simulink model "controller13_jumping"  (R2023a)
settings: Solver=FixedStepAuto  StartTime=0.0  StopTime=mdl.exe_time  RelTol=1e-3
values from neighbouring files (symbols this model uses):
  ctr2 = ctr    [s1_setup.m]    (also in step1_setup.m; step1_setup_v1.m)
  lut = gen_lut    [s1_setup.m]    (also in thrust2voltage_lut_20230809.mat = ; thrust2voltage_lut_20230829.mat = )
  mdl = make_model(mdl,rsim)    [s1_setup.m]    (also in setup_controller_with_functions.m = make_model(flight_time); step1_setup.m; step1_setup_v1.m = make_model(flight_time,rsim))
undefined symbols (not defined in the file or in its folder): Angle, Axis, DiscIntNeverNeededParam, rjsim, servo_config, Standard_Devices, UDP_Protocol, use_simulation
libraries: simulink x25, sldrtlib x9, robotcorelib x8, dspmathops x3, dspswit3 x2, shared6dofsys x2, dspfdesign x2, sharedtransform x1, sharedutil x1, matrix_library x1, shared6dof x1, simulink_extras x1
(part 3 of 3)

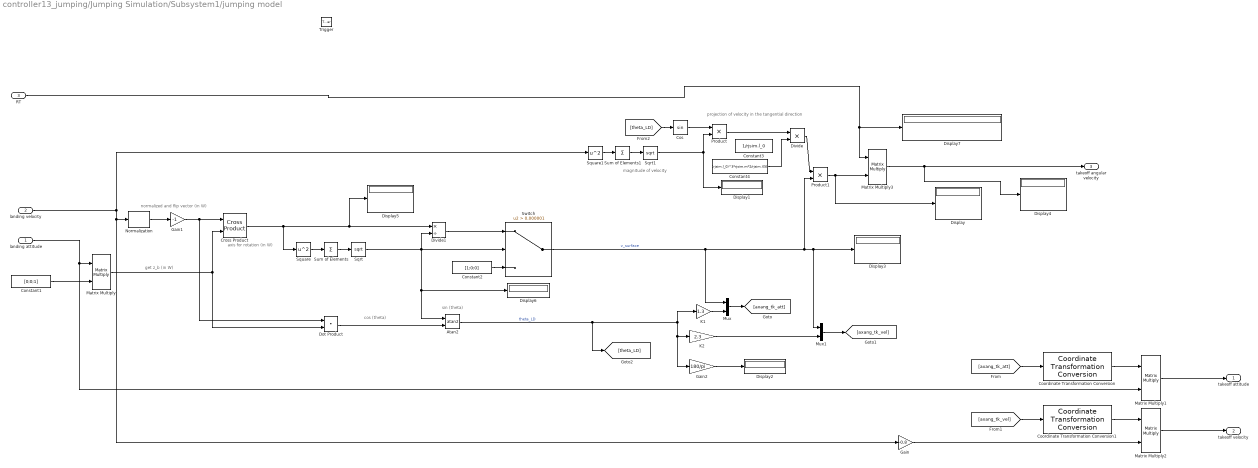
== system controller13_jumping/Jumping Simulation/Subsystem1/jumping model ==
  note: normalized and flip vector (in W)
  note: get z_b (in W)
  note: axis for rotation (in W)
  note: cos (theta)
  note: sin (theta)
  note: magnitude of velocity
  note: projection of velocity in the tangential direction
  landing attitude : Inport
  landing velocity : Inport  Port=2
  RT : Inport  Port=3
  Trigger : TriggerPort  VariantControl=(inherit)
  Atan2 : Trigonometry  Operator=atan2
  Constant1 : Constant  Value=[0;0;1]
  Constant2 : Constant  Value=[1;0;0]
  Constant3 : Constant  Value=1/rjsim.l_0
  Constant4 : Constant  Value=(rjsim.l_0)^3*rjsim.m*2/rjsim.I(5)
  Coordinate Transformation Conversion : robotcorelib/Coordinate Transformation Conversion  InputRepresentation=Axis-Angle  InputEulerSequence=ZYX  ShowTrVecInputPort=on  OutputRepresentation=Rotation Matrix  OutputEulerSequence=ZYX  ShowTrVecOutputPort=on  SimulateUsing=Interpreted execution
      settings: LibrarySourceBlock=navlib/Utilities/Coordinate Transformation Conversion
  Coordinate Transformation Conversion1 : robotcorelib/Coordinate Transformation Conversion  InputRepresentation=Axis-Angle  InputEulerSequence=ZYX  ShowTrVecInputPort=on  OutputRepresentation=Rotation Matrix  OutputEulerSequence=ZYX  ShowTrVecOutputPort=on  SimulateUsing=Interpreted execution
      settings: LibrarySourceBlock=navlib/Utilities/Coordinate Transformation Conversion
  Cos : Trigonometry
  Cross Product : matrix_library/Cross Product
  Display{,1..7} (8 alike) : Display
  Divide : Product  Inputs=**
  Divide1 : Product  Inputs=*/
  Dot Product : DotProduct  OutDataTypeStr=Inherit: Inherit via internal rule
  Gain : Gain  Gain=-0.8
  Gain1 : Gain  Gain=-1
  Gain2 : Gain  Gain=180/pi
  K1 : Gain  Gain=1.3
  K2 : Gain  Gain=2.3
  Matrix Multiply{,1..3} (4 alike) : Product  Multiplication=Matrix(*)
  Mux : Mux  Inputs=2
  Mux1 : Mux  Inputs=2
  Normalization : dspmathops/Normalization  NormType=Squared 2-norm  Bias=1e-10  NormOver=Each column  Dimension=1  roundingMode=Floor  overflowMode=off  accumDataTypeStr=Inherit: Same as product output  accumLastDataTypeStr=Inherit: Same as product output  outputDataTypeStr=Inherit: Same as product output  outputMin=[]  outputMax=[]  outputLastDataTypeStr=Inherit: Same as product output
  Product : Product
  Product1 : Product
  Sqrt : Sqrt
  Sqrt1 : Sqrt
  Square : Math  Operator=square
  Square1 : Math  Operator=square
  Sum of Elements : Sum  Inputs=+
  Sum of Elements1 : Sum  Inputs=+
  Switch : Switch  Criteria=u2 > Threshold  Threshold=0.000001  SaturateOnIntegerOverflow=off  InputSameDT=off
  takeoff attitude : Outport
  takeoff velocity : Outport  Port=2
  takeoff angular velocity : Outport  Port=3
  wires:
  landing velocity/1 -> Gain/1, Normalization/1, Square1/1
  landing attitude/1 -> Matrix Multiply1/2, Matrix Multiply/1
  Constant1/1 -> Matrix Multiply/2
  Normalization/1 -> Gain1/1
  Gain1/1 -> Dot Product/1, Cross Product/1
  Matrix Multiply/1 -> Dot Product/2, Cross Product/2
  Cross Product/1 -> Divide1/1, Display5/1, Square/1
  Square/1 -> Sum of Elements/1
  Sum of Elements/1 -> Sqrt/1
  Sqrt/1 -> Divide1/2, Atan2/1, Display6/1, Switch/2
  Constant2/1 -> Switch/3
  Dot Product/1 -> Atan2/2
  Atan2/1 -> [theta_LD], Gain2/1, K2/1, K1/1  "theta_LD"
  K1/1 -> Mux/2
  Mux/1 -> [axang_tk_att]
  Switch/1 -> Display3/1, Mux1/1, Product1/2, Mux/1  "v_surface"
  Mux1/1 -> [axang_tk_vel]
  K2/1 -> Mux1/2
  Matrix Multiply1/1 -> takeoff attitude/1
  [axang_tk_att] -> Coordinate Transformation Conversion/1
  Coordinate Transformation Conversion/1 -> Matrix Multiply1/1
  [axang_tk_vel] -> Coordinate Transformation Conversion1/1
  Coordinate Transformation Conversion1/1 -> Matrix Multiply2/1
  Gain/1 -> Matrix Multiply2/2
  Matrix Multiply2/1 -> takeoff velocity/1
  Square1/1 -> Sum of Elements1/1
  Sum of Elements1/1 -> Sqrt1/1
  [theta_LD] -> Cos/1
  Cos/1 -> Product/1
  Sqrt1/1 -> Display1/1, Product/2
  Product/1 -> Divide/1
  Divide/1 -> Product1/1
  Product1/1 -> Matrix Multiply3/2, Display/1
  Gain2/1 -> Display2/1
  Divide1/1 -> Switch/1
  RT/1 -> Matrix Multiply3/1, Display7/1
  Matrix Multiply3/1 -> Display4/1, takeoff angular velocity/1
  Constant4/1 -> Divide/2

== system controller13_jumping/Measurement manager 2/safety check system/landing condition ==
  z : Inport
  Add : Sum  Inputs=+--
  SaturatingRamp1 : DiscreteIntegrator  gainval=1  SampleTime=-1  UpperSaturationLimit=1  LowerSaturationLimit=0  ICPrevOutput=DiscIntNeverNeededParam  ICPrevScaledInput=DiscIntNeverNeededParam
  constant : Constant
  constant1 : Constant  Value=2
  constant2 : Constant  Value=mdl.i_delay
  landing_cond : MATLAB Function  TreatAsAtomicUnit=on  SystemSampleTime=mdl.T
  en : Outport
  wires:
  SaturatingRamp1/1 -> Add/1
  constant/1 -> SaturatingRamp1/1
  constant1/1 -> Add/2
  constant2/1 -> Add/3
  Add/1 -> landing_cond/2(time_cond)
  z/1 -> landing_cond/1(alt)
  landing_cond/1(en) -> en/1

== system controller13_jumping/Subsystem6/Subsystem4/If Action Subsystem ==
  In1 : Inport
  In2 : Inport  Port=2
  Action Port : ActionPort  ActionPortLabel=else
  Divide : Product  Inputs=*/
  Out1 : Outport
  wires:
  In1/1 -> Divide/1
  In2/1 -> Divide/2
  Divide/1 -> Out1/1

== system controller13_jumping/Subsystem6/Subsystem4/If Action Subsystem1 ==
  Action Port : ActionPort  ActionPortLabel=if(u1 == 0)
  Constant : Constant  Value=[0;0;0]
  Out1 : Outport
  wires:
  Constant/1 -> Out1/1

== system controller13_jumping/Subsystem6/Subsystem4/Triggered Subsystem ==
  In1 : Inport
  In2 : Inport  Port=2
  Trigger : TriggerPort  VariantControl=(inherit)
  Scope : Scope  NumInputPorts=2
  Timestamp : sldrtlib/Target Profiling/Timestamp
  Unit Delay : UnitDelay  SampleTime=-1  HasFrameUpgradeWarning=on
  Unit Delay1 : UnitDelay  SampleTime=-1  HasFrameUpgradeWarning=on
  Out1 : Outport
  Output : Outport  Port=2
  Output1 : Outport  Port=3
  Output2 : Outport  Port=4
  wires:
  Unit Delay/1 -> Output/1
  Unit Delay1/1 -> Scope/2, Output2/1
  In1/1 -> Unit Delay/1, Out1/1
  In2/1 -> Unit Delay1/1, Scope/1, Output1/1

== system controller13_jumping/Subsystem6/Subsystem5/If Action Subsystem ==
  In1 : Inport
  In2 : Inport  Port=2
  Action Port : ActionPort  ActionPortLabel=else
  Divide : Product  Inputs=*/
  Out1 : Outport
  wires:
  In1/1 -> Divide/1
  In2/1 -> Divide/2
  Divide/1 -> Out1/1

== system controller13_jumping/Subsystem6/Subsystem5/If Action Subsystem1 ==
  Action Port : ActionPort  ActionPortLabel=if(u1 == 0)
  Constant : Constant  Value=zeros(9,1)
  Out1 : Outport
  wires:
  Constant/1 -> Out1/1

== system controller13_jumping/Subsystem6/Subsystem5/Triggered Subsystem ==
  R : Inport
  In2 : Inport  Port=2
  Trigger : TriggerPort  VariantControl=(inherit)
  Scope : Scope  NumInputPorts=2
  Timestamp : sldrtlib/Target Profiling/Timestamp
  Unit Delay : UnitDelay  SampleTime=-1  HasFrameUpgradeWarning=on
  Unit Delay1 : UnitDelay  SampleTime=-1  HasFrameUpgradeWarning=on
  Out1 : Outport
  Output : Outport  Port=2
  Output1 : Outport  Port=3
  Output2 : Outport  Port=4
  wires:
  Unit Delay/1 -> Output/1
  Unit Delay1/1 -> Scope/2, Output2/1
  R/1 -> Unit Delay/1, Out1/1
  In2/1 -> Unit Delay1/1, Scope/1, Output1/1

== system controller13_jumping/signal generator1/Bias_Signal/AveragedBias ==
  note: To avoid having signal "jump",
      | we want SMOOTH transitions
      | in frequency (i.e., a weighted sum
      | of current freq and freq some delta t ago)
  note: time constant = 0.002sec
  In1 : Inport
  Discrete Transfer Fcn : DiscreteTransferFcn  Commented=through  Numerator=[0.05]  Denominator=[1 -.95]
  Out1 : Outport
  wires:
  In1/1 -> Discrete Transfer Fcn/1
  Discrete Transfer Fcn/1 -> Out1/1

== system controller13_jumping/signal generator1/Bias_Signal/SIgnalForRamp_binary ==
  note: Should output 1 or -1,
      | so signal ramps UP to 1
      | or DOWN to 0.
  In1 : Inport
  Add : Sum  Inputs=+-
  Compare To Zero : simulink/Logic and Bit Operations/Compare To Zero  relop=>  OutDataTypeStr=uint8  ZeroCross=off
  Constant : Constant
  Data Type Conversion : DataTypeConversion  OutDataTypeStr=double  SaturateOnIntegerOverflow=off  RndMeth=Floor
  Gain : Gain  Gain=2
  Out1 : Outport
  wires:
  In1/1 -> Compare To Zero/1
  Compare To Zero/1 -> Data Type Conversion/1
  Gain/1 -> Add/1
  Constant/1 -> Add/2
  Add/1 -> Out1/1
  Data Type Conversion/1 -> Gain/1

== system controller13_jumping/signal generator1/Drive_Signal1/AveragedAmp_filtered ==
  note: To avoid having signal "jump",
      | we want SMOOTH transitions
      | in frequency (i.e., a weighted sum
      | of current freq and freq some delta t ago)
  note: time constant 0.002sec
      | for 10kHz samping
  In1 : Inport
  Discrete Transfer Fcn : DiscreteTransferFcn  Commented=through  Numerator=[0.05]  Denominator=[1 -.95]
  Out1 : Outport
  wires:
  In1/1 -> Discrete Transfer Fcn/1
  Discrete Transfer Fcn/1 -> Out1/1

== system controller13_jumping/signal generator1/Drive_Signal1/AveragedOffset_filtered ==
  note: To avoid having signal "jump",
      | we want SMOOTH transitions
      | in frequency (i.e., a weighted sum
      | of current freq and freq some delta t ago)
  note: c
  note: time constant 0.02sec
      | for 10kHz samping
  In1 : Inport
  Discrete Transfer Fcn : DiscreteTransferFcn  Commented=through  Numerator=[0.05]  Denominator=[1 -.95]
  Out1 : Outport
  wires:
  In1/1 -> Discrete Transfer Fcn/1
  Discrete Transfer Fcn/1 -> Out1/1

== system controller13_jumping/signal generator1/Drive_Signal1/AveragedTau_filtered ==
  note: To avoid having signal "jump",
      | we want SMOOTH transitions
      | in frequency (i.e., a weighted sum
      | of current freq and freq some delta t ago)
  note: time constant 0.002sec
      | for 10kHz samping
  In1 : Inport
  Discrete Transfer Fcn : DiscreteTransferFcn  Numerator=[0.05]  Denominator=[1, -0.95]
  Out1 : Outport
  wires:
  In1/1 -> Discrete Transfer Fcn/1
  Discrete Transfer Fcn/1 -> Out1/1

== system controller13_jumping/signal generator1/Drive_Signal1/SignalForRamp_binary ==
  note: Should output 1 or -1,
      | so signal ramps UP to 1
      | or DOWN to 0.
  In1 : Inport
  Add : Sum  Inputs=+-
  Compare To Zero : simulink/Logic and Bit Operations/Compare To Zero  relop=>  OutDataTypeStr=uint8  ZeroCross=off
  Constant : Constant
  Data Type Conversion : DataTypeConversion  OutDataTypeStr=double  SaturateOnIntegerOverflow=off  RndMeth=Floor
  Gain : Gain  Gain=2
  Out1 : Outport
  wires:
  In1/1 -> Compare To Zero/1
  Compare To Zero/1 -> Data Type Conversion/1
  Gain/1 -> Add/1
  Constant/1 -> Add/2
  Add/1 -> Out1/1
  Data Type Conversion/1 -> Gain/1

== system controller13_jumping/signal generator1/Drive_Signal1/SignalForSin_binary ==
  note: We want this to stay "high" for 1
      | second after the actual "enable"
      | is turned off...
  In1 : Inport
  Compare To Zero : simulink/Logic and Bit Operations/Compare To Zero  relop=>  OutDataTypeStr=uint8  ZeroCross=off
  Data Type Conversion : DataTypeConversion  OutDataTypeStr=double  SaturateOnIntegerOverflow=off  RndMeth=Floor
  Out1 : Outport
  wires:
  In1/1 -> Compare To Zero/1
  Compare To Zero/1 -> Data Type Conversion/1
  Data Type Conversion/1 -> Out1/1

== system controller13_jumping/signal generator1/Drive_Signal1/Subsystem ==
  note: positive value pushes the left wing forward
  split cycle mu : Inport
  In2 : Inport  Port=2
  1-mu : Sum  Inputs=+-
  2f : Gain  Gain=2
  2nd harmonic : Trigonometry  OutputSignalType=real
  2pi : Gain  Gain=2*pi
  Abs1 : Abs  SaturateOnIntegerOverflow=off
  Add : Sum
  Constant : Constant
  combined sines : Sum
  deg to rad : Gain  Gain=pi/180
  f : Gain  Gain=-1
  first harmonic : Trigonometry  OutputSignalType=real
  omega*t : DiscreteIntegrator  SampleTime=-1  ICPrevOutput=DiscIntNeverNeededParam  ICPrevScaledInput=DiscIntNeverNeededParam
  phase offset : Constant  Value=0
  signal with gain1 : Product  RndMeth=Zero
  signal with gain2 : Product  RndMeth=Zero
  split cycle signal : Outport
  wires:
  2f/1 -> 2nd harmonic/1
  first harmonic/1 -> signal with gain1/2
  Constant/1 -> 1-mu/1
  split cycle mu/1 -> f/1, Abs1/1
  1-mu/1 -> signal with gain1/1
  2nd harmonic/1 -> signal with gain2/2
  signal with gain1/1 -> combined sines/1
  signal with gain2/1 -> combined sines/2
  combined sines/1 -> split cycle signal/1
  f/1 -> signal with gain2/1
  Abs1/1 -> 1-mu/2
  In2/1 -> 2pi/1
  2pi/1 -> omega*t/1
  omega*t/1 -> Add/2
  Add/1 -> first harmonic/1, 2f/1
  phase offset/1 -> deg to rad/1
  deg to rad/1 -> Add/1

== system controller13_jumping/signal generator1/Drive_Signal2/AveragedAmp_filtered ==
  note: To avoid having signal "jump",
      | we want SMOOTH transitions
      | in frequency (i.e., a weighted sum
      | of current freq and freq some delta t ago)
  note: time constant 0.002sec
      | for 10kHz samping
  In1 : Inport
  Discrete Transfer Fcn : DiscreteTransferFcn  Numerator=[0.05]  Denominator=[1 -.95]
  Out1 : Outport
  wires:
  In1/1 -> Discrete Transfer Fcn/1
  Discrete Transfer Fcn/1 -> Out1/1

== system controller13_jumping/signal generator1/Drive_Signal2/AveragedOffset_filtered ==
  note: To avoid having signal "jump",
      | we want SMOOTH transitions
      | in frequency (i.e., a weighted sum
      | of current freq and freq some delta t ago)
  note: c
  note: time constant 0.02sec
      | for 10kHz samping
  In1 : Inport
  Discrete Transfer Fcn : DiscreteTransferFcn  Numerator=[0.05]  Denominator=[1 -.95]
  Out1 : Outport
  wires:
  In1/1 -> Discrete Transfer Fcn/1
  Discrete Transfer Fcn/1 -> Out1/1

== system controller13_jumping/signal generator1/Drive_Signal2/AveragedTau_filtered ==
  note: To avoid having signal "jump",
      | we want SMOOTH transitions
      | in frequency (i.e., a weighted sum
      | of current freq and freq some delta t ago)
  note: time constant 0.002sec
      | for 10kHz samping
  In1 : Inport
  Discrete Transfer Fcn : DiscreteTransferFcn  Numerator=[0.05]  Denominator=[1, -0.95]
  Out1 : Outport
  wires:
  In1/1 -> Discrete Transfer Fcn/1
  Discrete Transfer Fcn/1 -> Out1/1

== system controller13_jumping/signal generator1/Drive_Signal2/SignalForRamp_binary ==
  note: Should output 1 or -1,
      | so signal ramps UP to 1
      | or DOWN to 0.
  In1 : Inport
  Add : Sum  Inputs=+-
  Compare To Zero : simulink/Logic and Bit Operations/Compare To Zero  relop=>  OutDataTypeStr=uint8  ZeroCross=off
  Constant : Constant
  Data Type Conversion : DataTypeConversion  OutDataTypeStr=double  SaturateOnIntegerOverflow=off  RndMeth=Floor
  Gain : Gain  Gain=2
  Out1 : Outport
  wires:
  In1/1 -> Compare To Zero/1
  Compare To Zero/1 -> Data Type Conversion/1
  Gain/1 -> Add/1
  Constant/1 -> Add/2
  Add/1 -> Out1/1
  Data Type Conversion/1 -> Gain/1

== system controller13_jumping/signal generator1/Drive_Signal2/SignalForSin_binary ==
  note: We want this to stay "high" for 1
      | second after the actual "enable"
      | is turned off...
  In1 : Inport
  Compare To Zero : simulink/Logic and Bit Operations/Compare To Zero  relop=>  OutDataTypeStr=uint8  ZeroCross=off
  Data Type Conversion : DataTypeConversion  OutDataTypeStr=double  SaturateOnIntegerOverflow=off  RndMeth=Floor
  Out1 : Outport
  wires:
  In1/1 -> Compare To Zero/1
  Compare To Zero/1 -> Data Type Conversion/1
  Data Type Conversion/1 -> Out1/1

== system controller13_jumping/signal generator1/Drive_Signal2/Subsystem ==
  note: positive value pushes the left wing forward
  split cycle mu : Inport
  In2 : Inport  Port=2
  1-mu : Sum  Inputs=+-
  2f : Gain  Gain=2
  2nd harmonic : Trigonometry  OutputSignalType=real
  2pi : Gain  Gain=2*pi
  Abs1 : Abs  SaturateOnIntegerOverflow=off
  Add : Sum
  Constant : Constant
  combined sines : Sum
  deg to rad : Gain  Gain=pi/180
  f : Gain  Gain=-1
  first harmonic : Trigonometry  OutputSignalType=real
  omega*t : DiscreteIntegrator  SampleTime=-1  ICPrevOutput=DiscIntNeverNeededParam  ICPrevScaledInput=DiscIntNeverNeededParam
  phase offset : Constant  Value=0
  signal with gain1 : Product  RndMeth=Zero
  signal with gain2 : Product  RndMeth=Zero
  split cycle signal : Outport
  wires:
  2f/1 -> 2nd harmonic/1
  first harmonic/1 -> signal with gain1/2
  Constant/1 -> 1-mu/1
  split cycle mu/1 -> f/1, Abs1/1
  1-mu/1 -> signal with gain1/1
  2nd harmonic/1 -> signal with gain2/2
  signal with gain1/1 -> combined sines/1
  signal with gain2/1 -> combined sines/2
  combined sines/1 -> split cycle signal/1
  f/1 -> signal with gain2/1
  Abs1/1 -> 1-mu/2
  In2/1 -> 2pi/1
  2pi/1 -> omega*t/1
  omega*t/1 -> Add/2
  Add/1 -> first harmonic/1, 2f/1
  phase offset/1 -> deg to rad/1
  deg to rad/1 -> Add/1

== system controller13_jumping/signal generator1/Drive_Signal3/AveragedAmp_filtered ==
  note: To avoid having signal "jump",
      | we want SMOOTH transitions
      | in frequency (i.e., a weighted sum
      | of current freq and freq some delta t ago)
  note: time constant 0.002sec
      | for 10kHz samping
  In1 : Inport
  Discrete Transfer Fcn : DiscreteTransferFcn  Numerator=[0.05]  Denominator=[1 -.95]
  Out1 : Outport
  wires:
  In1/1 -> Discrete Transfer Fcn/1
  Discrete Transfer Fcn/1 -> Out1/1

== system controller13_jumping/signal generator1/Drive_Signal3/AveragedOffset_filtered ==
  note: To avoid having signal "jump",
      | we want SMOOTH transitions
      | in frequency (i.e., a weighted sum
      | of current freq and freq some delta t ago)
  note: c
  note: time constant 0.02sec
      | for 10kHz samping
  In1 : Inport
  Discrete Transfer Fcn : DiscreteTransferFcn  Numerator=[0.05]  Denominator=[1 -.95]
  Out1 : Outport
  wires:
  In1/1 -> Discrete Transfer Fcn/1
  Discrete Transfer Fcn/1 -> Out1/1

== system controller13_jumping/signal generator1/Drive_Signal3/AveragedTau_filtered ==
  note: To avoid having signal "jump",
      | we want SMOOTH transitions
      | in frequency (i.e., a weighted sum
      | of current freq and freq some delta t ago)
  note: time constant 0.002sec
      | for 10kHz samping
  In1 : Inport
  Discrete Transfer Fcn : DiscreteTransferFcn  Numerator=[0.05]  Denominator=[1 -.95]
  Out1 : Outport
  wires:
  In1/1 -> Discrete Transfer Fcn/1
  Discrete Transfer Fcn/1 -> Out1/1

== system controller13_jumping/signal generator1/Drive_Signal3/SignalForRamp_binary ==
  note: Should output 1 or -1,
      | so signal ramps UP to 1
      | or DOWN to 0.
  In1 : Inport
  Add : Sum  Inputs=+-
  Compare To Zero : simulink/Logic and Bit Operations/Compare To Zero  relop=>  OutDataTypeStr=uint8  ZeroCross=off
  Constant : Constant
  Data Type Conversion : DataTypeConversion  OutDataTypeStr=double  SaturateOnIntegerOverflow=off  RndMeth=Floor
  Gain : Gain  Gain=2
  Out1 : Outport
  wires:
  In1/1 -> Compare To Zero/1
  Compare To Zero/1 -> Data Type Conversion/1
  Gain/1 -> Add/1
  Constant/1 -> Add/2
  Add/1 -> Out1/1
  Data Type Conversion/1 -> Gain/1

== system controller13_jumping/signal generator1/Drive_Signal3/SignalForSin_binary ==
  note: We want this to stay "high" for 1
      | second after the actual "enable"
      | is turned off...
  In1 : Inport
  Compare To Zero : simulink/Logic and Bit Operations/Compare To Zero  relop=>  OutDataTypeStr=uint8  ZeroCross=off
  Data Type Conversion : DataTypeConversion  OutDataTypeStr=double  SaturateOnIntegerOverflow=off  RndMeth=Floor
  Out1 : Outport
  wires:
  In1/1 -> Compare To Zero/1
  Compare To Zero/1 -> Data Type Conversion/1
  Data Type Conversion/1 -> Out1/1

== system controller13_jumping/signal generator1/Drive_Signal3/Subsystem ==
  split cycle mu : Inport
  In2 : Inport  Port=2
  1-mu : Sum  Inputs=+-
  2f : Gain  Gain=2
  2nd harmonic : Trigonometry  OutputSignalType=real
  2pi : Gain  Gain=2*pi
  Abs1 : Abs  SaturateOnIntegerOverflow=off
  Constant : Constant
  SmoothClock : DiscreteIntegrator  SampleTime=-1  ICPrevOutput=DiscIntNeverNeededParam  ICPrevScaledInput=DiscIntNeverNeededParam
  combined sines : Sum
  f : Gain
  first harmonic : Trigonometry  OutputSignalType=real
  signal with gain1 : Product  RndMeth=Zero
  signal with gain2 : Product  RndMeth=Zero
  split cycle signal : Outport
  wires:
  SmoothClock/1 -> first harmonic/1, 2f/1
  2f/1 -> 2nd harmonic/1
  2pi/1 -> SmoothClock/1
  first harmonic/1 -> signal with gain1/2
  Constant/1 -> 1-mu/1
  split cycle mu/1 -> f/1, Abs1/1
  1-mu/1 -> signal with gain1/1
  2nd harmonic/1 -> signal with gain2/2
  signal with gain1/1 -> combined sines/1
  signal with gain2/1 -> combined sines/2
  combined sines/1 -> split cycle signal/1
  In2/1 -> 2pi/1
  f/1 -> signal with gain2/1
  Abs1/1 -> 1-mu/2

== system controller13_jumping/signal generator1/Drive_Signal4/AveragedAmp_filtered ==
  note: To avoid having signal "jump",
      | we want SMOOTH transitions
      | in frequency (i.e., a weighted sum
      | of current freq and freq some delta t ago)
  note: time constant 0.002sec
      | for 10kHz samping
  In1 : Inport
  Discrete Transfer Fcn : DiscreteTransferFcn  Commented=through  Numerator=[0.05]  Denominator=[1 -.95]
  Out1 : Outport
  wires:
  In1/1 -> Discrete Transfer Fcn/1
  Discrete Transfer Fcn/1 -> Out1/1

== system controller13_jumping/signal generator1/Drive_Signal4/AveragedOffset_filtered ==
  note: To avoid having signal "jump",
      | we want SMOOTH transitions
      | in frequency (i.e., a weighted sum
      | of current freq and freq some delta t ago)
  note: c
  note: time constant 0.02sec
      | for 10kHz samping
  In1 : Inport
  Discrete Transfer Fcn : DiscreteTransferFcn  Commented=through  Numerator=[0.05]  Denominator=[1 -.95]
  Out1 : Outport
  wires:
  In1/1 -> Discrete Transfer Fcn/1
  Discrete Transfer Fcn/1 -> Out1/1

== system controller13_jumping/signal generator1/Drive_Signal4/AveragedTau_filtered ==
  note: To avoid having signal "jump",
      | we want SMOOTH transitions
      | in frequency (i.e., a weighted sum
      | of current freq and freq some delta t ago)
  note: time constant 0.002sec
      | for 10kHz samping
  In1 : Inport
  Discrete Transfer Fcn : DiscreteTransferFcn  Numerator=[0.05]  Denominator=[1, -0.95]
  Out1 : Outport
  wires:
  In1/1 -> Discrete Transfer Fcn/1
  Discrete Transfer Fcn/1 -> Out1/1

== system controller13_jumping/signal generator1/Drive_Signal4/SignalForRamp_binary ==
  note: Should output 1 or -1,
      | so signal ramps UP to 1
      | or DOWN to 0.
  In1 : Inport
  Add : Sum  Inputs=+-
  Compare To Zero : simulink/Logic and Bit Operations/Compare To Zero  relop=>  OutDataTypeStr=uint8  ZeroCross=off
  Constant : Constant
  Data Type Conversion : DataTypeConversion  OutDataTypeStr=double  SaturateOnIntegerOverflow=off  RndMeth=Floor
  Gain : Gain  Gain=2
  Out1 : Outport
  wires:
  In1/1 -> Compare To Zero/1
  Compare To Zero/1 -> Data Type Conversion/1
  Gain/1 -> Add/1
  Constant/1 -> Add/2
  Add/1 -> Out1/1
  Data Type Conversion/1 -> Gain/1

== system controller13_jumping/signal generator1/Drive_Signal4/SignalForSin_binary ==
  note: We want this to stay "high" for 1
      | second after the actual "enable"
      | is turned off...
  In1 : Inport
  Compare To Zero : simulink/Logic and Bit Operations/Compare To Zero  relop=>  OutDataTypeStr=uint8  ZeroCross=off
  Data Type Conversion : DataTypeConversion  OutDataTypeStr=double  SaturateOnIntegerOverflow=off  RndMeth=Floor
  Out1 : Outport
  wires:
  In1/1 -> Compare To Zero/1
  Compare To Zero/1 -> Data Type Conversion/1
  Data Type Conversion/1 -> Out1/1

== system controller13_jumping/signal generator1/Drive_Signal4/Subsystem ==
  note: positive value pushes the left wing forward
  split cycle mu : Inport
  In2 : Inport  Port=2
  1-mu : Sum  Inputs=+-
  2f : Gain  Gain=2
  2nd harmonic : Trigonometry  OutputSignalType=real
  2pi : Gain  Gain=2*pi
  Abs1 : Abs  SaturateOnIntegerOverflow=off
  Add : Sum
  Constant : Constant
  combined sines : Sum
  deg to rad : Gain  Gain=pi/180
  f : Gain  Gain=-1
  first harmonic : Trigonometry  OutputSignalType=real
  omega*t : DiscreteIntegrator  SampleTime=-1  ICPrevOutput=DiscIntNeverNeededParam  ICPrevScaledInput=DiscIntNeverNeededParam
  phase offset : Constant  Value=0
  signal with gain1 : Product  RndMeth=Zero
  signal with gain2 : Product  RndMeth=Zero
  split cycle signal : Outport
  wires:
  2f/1 -> 2nd harmonic/1
  first harmonic/1 -> signal with gain1/2
  Constant/1 -> 1-mu/1
  split cycle mu/1 -> f/1, Abs1/1
  1-mu/1 -> signal with gain1/1
  2nd harmonic/1 -> signal with gain2/2
  signal with gain1/1 -> combined sines/1
  signal with gain2/1 -> combined sines/2
  combined sines/1 -> split cycle signal/1
  f/1 -> signal with gain2/1
  Abs1/1 -> 1-mu/2
  In2/1 -> 2pi/1
  2pi/1 -> omega*t/1
  omega*t/1 -> Add/2
  Add/1 -> first harmonic/1, 2f/1
  phase offset/1 -> deg to rad/1
  deg to rad/1 -> Add/1

== system controller13_jumping/signal generator1/signal generator 1/SignalForRamp_binary ==
  note: Should output 1 or -1,
      | so signal ramps UP to 1
      | or DOWN to 0.
  EnableSignal : Inport
  Add : Sum  Inputs=+-
  Compare To Zero : simulink/Logic and Bit Operations/Compare To Zero  relop=>  OutDataTypeStr=uint8  ZeroCross=off
  Constant : Constant
  Data Type Conversion : DataTypeConversion  OutDataTypeStr=double  SaturateOnIntegerOverflow=off  RndMeth=Floor
  Gain : Gain  Gain=2
  Out1 : Outport
  wires:
  EnableSignal/1 -> Compare To Zero/1
  Compare To Zero/1 -> Data Type Conversion/1
  Gain/1 -> Add/1
  Constant/1 -> Add/2
  Add/1 -> Out1/1
  Data Type Conversion/1 -> Gain/1

== system controller13_jumping/signal generator1/signal generator 1/SignalSaturationLimit4 ==
  Max : Inport
  SignalRaw : Inport  Port=2
  MaxOf : MinMax  Function=max  Inputs=2
  MinOf : MinMax  Inputs=2
  ground : Constant
  SignalSatd : Outport
  wires:
  SignalRaw/1 -> MinOf/2
  MinOf/1 -> MaxOf/1
  MaxOf/1 -> SignalSatd/1
  Max/1 -> MinOf/1
  ground/1 -> MaxOf/2

== system controller13_jumping/signal generator1/signal generator 1/get max voltage ==
  note: time constant = 0.002sec
  QuasiEnable : Inport
  max voltage : Inport  Port=2
  Product : Product  RndMeth=Zero
  SIgnalForRamp_binary : Subsystem
  SaturatingRamp : DiscreteIntegrator  gainval=100  SampleTime=-1  LimitOutput=on  UpperSaturationLimit=1  LowerSaturationLimit=0  ICPrevOutput=DiscIntNeverNeededParam  ICPrevScaledInput=DiscIntNeverNeededParam
  max signa; : Outport
  wires:
  Product/1 -> max signa;/1
  max voltage/1 -> Product/2
  QuasiEnable/1 -> SIgnalForRamp_binary/1(In1)
  SIgnalForRamp_binary/1(Out1) -> SaturatingRamp/1
  SaturatingRamp/1 -> Product/1

== system controller13_jumping/signal generator1/signal generator 2/SignalForRamp_binary ==
  note: Should output 1 or -1,
      | so signal ramps UP to 1
      | or DOWN to 0.
  EnableSignal : Inport
  Add : Sum  Inputs=+-
  Compare To Zero : simulink/Logic and Bit Operations/Compare To Zero  relop=>  OutDataTypeStr=uint8  ZeroCross=off
  Constant : Constant
  Data Type Conversion : DataTypeConversion  OutDataTypeStr=double  SaturateOnIntegerOverflow=off  RndMeth=Floor
  Gain : Gain  Gain=2
  Out1 : Outport
  wires:
  EnableSignal/1 -> Compare To Zero/1
  Compare To Zero/1 -> Data Type Conversion/1
  Gain/1 -> Add/1
  Constant/1 -> Add/2
  Add/1 -> Out1/1
  Data Type Conversion/1 -> Gain/1

== system controller13_jumping/signal generator1/signal generator 2/SignalSaturationLimit4 ==
  Max : Inport
  SignalRaw : Inport  Port=2
  MaxOf : MinMax  Function=max  Inputs=2
  MinOf : MinMax  Inputs=2
  ground : Constant
  SignalSatd : Outport
  wires:
  SignalRaw/1 -> MinOf/2
  MinOf/1 -> MaxOf/1
  MaxOf/1 -> SignalSatd/1
  Max/1 -> MinOf/1
  ground/1 -> MaxOf/2

== system controller13_jumping/signal generator1/signal generator 2/get max voltage ==
  note: time constant = 0.002sec
  QuasiEnable : Inport
  max voltage : Inport  Port=2
  Product : Product  RndMeth=Zero
  SIgnalForRamp_binary : Subsystem
  SaturatingRamp : DiscreteIntegrator  gainval=100  SampleTime=-1  LimitOutput=on  UpperSaturationLimit=1  LowerSaturationLimit=0  ICPrevOutput=DiscIntNeverNeededParam  ICPrevScaledInput=DiscIntNeverNeededParam
  max signa; : Outport
  wires:
  Product/1 -> max signa;/1
  max voltage/1 -> Product/2
  QuasiEnable/1 -> SIgnalForRamp_binary/1(In1)
  SIgnalForRamp_binary/1(Out1) -> SaturatingRamp/1
  SaturatingRamp/1 -> Product/1

== system controller13_jumping/signal generator1/signal generator 3/SignalForRamp_binary ==
  note: Should output 1 or -1,
      | so signal ramps UP to 1
      | or DOWN to 0.
  EnableSignal : Inport
  Add : Sum  Inputs=+-
  Compare To Zero : simulink/Logic and Bit Operations/Compare To Zero  relop=>  OutDataTypeStr=uint8  ZeroCross=off
  Constant : Constant
  Data Type Conversion : DataTypeConversion  OutDataTypeStr=double  SaturateOnIntegerOverflow=off  RndMeth=Floor
  Gain : Gain  Gain=2
  Out1 : Outport
  wires:
  EnableSignal/1 -> Compare To Zero/1
  Compare To Zero/1 -> Data Type Conversion/1
  Gain/1 -> Add/1
  Constant/1 -> Add/2
  Add/1 -> Out1/1
  Data Type Conversion/1 -> Gain/1

== system controller13_jumping/signal generator1/signal generator 3/SignalSaturationLimit4 ==
  Max : Inport
  SignalRaw : Inport  Port=2
  MaxOf : MinMax  Function=max  Inputs=2
  MinOf : MinMax  Inputs=2
  ground : Constant
  SignalSatd : Outport
  wires:
  SignalRaw/1 -> MinOf/2
  MinOf/1 -> MaxOf/1
  MaxOf/1 -> SignalSatd/1
  Max/1 -> MinOf/1
  ground/1 -> MaxOf/2

== system controller13_jumping/signal generator1/signal generator 3/get max voltage ==
  note: time constant = 0.002sec
  QuasiEnable : Inport
  max voltage : Inport  Port=2
  Product : Product  RndMeth=Zero
  SIgnalForRamp_binary : Subsystem
  SaturatingRamp : DiscreteIntegrator  gainval=100  SampleTime=-1  LimitOutput=on  UpperSaturationLimit=1  LowerSaturationLimit=0  ICPrevOutput=DiscIntNeverNeededParam  ICPrevScaledInput=DiscIntNeverNeededParam
  max signa; : Outport
  wires:
  Product/1 -> max signa;/1
  max voltage/1 -> Product/2
  QuasiEnable/1 -> SIgnalForRamp_binary/1(In1)
  SIgnalForRamp_binary/1(Out1) -> SaturatingRamp/1
  SaturatingRamp/1 -> Product/1

== system controller13_jumping/signal generator1/signal generator 4/SignalForRamp_binary ==
  note: Should output 1 or -1,
      | so signal ramps UP to 1
      | or DOWN to 0.
  EnableSignal : Inport
  Add : Sum  Inputs=+-
  Compare To Zero : simulink/Logic and Bit Operations/Compare To Zero  relop=>  OutDataTypeStr=uint8  ZeroCross=off
  Constant : Constant
  Data Type Conversion : DataTypeConversion  OutDataTypeStr=double  SaturateOnIntegerOverflow=off  RndMeth=Floor
  Gain : Gain  Gain=2
  Out1 : Outport
  wires:
  EnableSignal/1 -> Compare To Zero/1
  Compare To Zero/1 -> Data Type Conversion/1
  Gain/1 -> Add/1
  Constant/1 -> Add/2
  Add/1 -> Out1/1
  Data Type Conversion/1 -> Gain/1

== system controller13_jumping/signal generator1/signal generator 4/SignalSaturationLimit4 ==
  Max : Inport
  SignalRaw : Inport  Port=2
  MaxOf : MinMax  Function=max  Inputs=2
  MinOf : MinMax  Inputs=2
  ground : Constant
  SignalSatd : Outport
  wires:
  SignalRaw/1 -> MinOf/2
  MinOf/1 -> MaxOf/1
  MaxOf/1 -> SignalSatd/1
  Max/1 -> MinOf/1
  ground/1 -> MaxOf/2

== system controller13_jumping/signal generator1/signal generator 4/get max voltage ==
  note: time constant = 0.002sec
  QuasiEnable : Inport
  max voltage : Inport  Port=2
  Product : Product  RndMeth=Zero
  SIgnalForRamp_binary : Subsystem
  SaturatingRamp : DiscreteIntegrator  gainval=100  SampleTime=-1  LimitOutput=on  UpperSaturationLimit=1  LowerSaturationLimit=0  ICPrevOutput=DiscIntNeverNeededParam  ICPrevScaledInput=DiscIntNeverNeededParam
  max signa; : Outport
  wires:
  Product/1 -> max signa;/1
  max voltage/1 -> Product/2
  QuasiEnable/1 -> SIgnalForRamp_binary/1(In1)
  SIgnalForRamp_binary/1(Out1) -> SaturatingRamp/1
  SaturatingRamp/1 -> Product/1

== system controller13_jumping/signal generator1/signal generator 1/get max voltage/SIgnalForRamp_binary ==
  note: Should output 1 or -1,
      | so signal ramps UP to 1
      | or DOWN to 0.
  In1 : Inport
  Add : Sum  Inputs=+-
  Compare To Zero : simulink/Logic and Bit Operations/Compare To Zero  relop=>  OutDataTypeStr=uint8  ZeroCross=off
  Constant : Constant
  Data Type Conversion : DataTypeConversion  OutDataTypeStr=double  SaturateOnIntegerOverflow=off  RndMeth=Floor
  Gain : Gain  Gain=2
  Out1 : Outport
  wires:
  In1/1 -> Compare To Zero/1
  Compare To Zero/1 -> Data Type Conversion/1
  Gain/1 -> Add/1
  Constant/1 -> Add/2
  Add/1 -> Out1/1
  Data Type Conversion/1 -> Gain/1

== system controller13_jumping/signal generator1/signal generator 2/get max voltage/SIgnalForRamp_binary ==
  note: Should output 1 or -1,
      | so signal ramps UP to 1
      | or DOWN to 0.
  In1 : Inport
  Add : Sum  Inputs=+-
  Compare To Zero : simulink/Logic and Bit Operations/Compare To Zero  relop=>  OutDataTypeStr=uint8  ZeroCross=off
  Constant : Constant
  Data Type Conversion : DataTypeConversion  OutDataTypeStr=double  SaturateOnIntegerOverflow=off  RndMeth=Floor
  Gain : Gain  Gain=2
  Out1 : Outport
  wires:
  In1/1 -> Compare To Zero/1
  Compare To Zero/1 -> Data Type Conversion/1
  Gain/1 -> Add/1
  Constant/1 -> Add/2
  Add/1 -> Out1/1
  Data Type Conversion/1 -> Gain/1

== system controller13_jumping/signal generator1/signal generator 3/get max voltage/SIgnalForRamp_binary ==
  note: Should output 1 or -1,
      | so signal ramps UP to 1
      | or DOWN to 0.
  In1 : Inport
  Add : Sum  Inputs=+-
  Compare To Zero : simulink/Logic and Bit Operations/Compare To Zero  relop=>  OutDataTypeStr=uint8  ZeroCross=off
  Constant : Constant
  Data Type Conversion : DataTypeConversion  OutDataTypeStr=double  SaturateOnIntegerOverflow=off  RndMeth=Floor
  Gain : Gain  Gain=2
  Out1 : Outport
  wires:
  In1/1 -> Compare To Zero/1
  Compare To Zero/1 -> Data Type Conversion/1
  Gain/1 -> Add/1
  Constant/1 -> Add/2
  Add/1 -> Out1/1
  Data Type Conversion/1 -> Gain/1

== system controller13_jumping/signal generator1/signal generator 4/get max voltage/SIgnalForRamp_binary ==
  note: Should output 1 or -1,
      | so signal ramps UP to 1
      | or DOWN to 0.
  In1 : Inport
  Add : Sum  Inputs=+-
  Compare To Zero : simulink/Logic and Bit Operations/Compare To Zero  relop=>  OutDataTypeStr=uint8  ZeroCross=off
  Constant : Constant
  Data Type Conversion : DataTypeConversion  OutDataTypeStr=double  SaturateOnIntegerOverflow=off  RndMeth=Floor
  Gain : Gain  Gain=2
  Out1 : Outport
  wires:
  In1/1 -> Compare To Zero/1
  Compare To Zero/1 -> Data Type Conversion/1
  Gain/1 -> Add/1
  Constant/1 -> Add/2
  Add/1 -> Out1/1
  Data Type Conversion/1 -> Gain/1

== matlab function controller13_jumping/landing attitude controller/landing_state_predictiction ==
  data: p_dot_landing output; time input; p input; p_landing output; p_dot input; g input; leg_length input; landing_time_stamp output
function [p_dot_landing, p_landing, landing_time_stamp]= fcn(time, p, p_dot, g, leg_length)

% safety
temp = (p_dot(3)^2/g + 2*(p(3)-leg_length))/g;
if temp <= 0
    t_total = 0.00001;
else
    t_total = p_dot(3)/g + ((p_dot(3)^2/g + 2*(p(3)-leg_length))/g)^(1/2);
end


landing_time_stamp = time + t_total;

x_landing = p(1) + p_dot(1) * t_total;
y_landing = p(2) + p_dot(2) * t_total;
z_landing = p(3) + p_dot(3) * t_total - 0.5 * g * t_total * t_total;

x_landing_dot = p_dot(1);
y_landing_dot = p_dot(2);
z_landing_dot = p_dot(3) - g * t_total;

p_landing = [x_landing; y_landing; z_landing];
p_dot_landing = [x_landing_dot; y_landing_dot; z_landing_dot];

return;
end

== matlab function controller13_jumping/Measurement manager 2/MATLAB Function ==
  data: keep_flying input; landing_in input; landing_out output size=1; cum_in input; cum_out output size=1; ctr2 parameter; mdl parameter
function [landing_out, cum_out] = fcn(keep_flying, landing_in, cum_in, ctr2, mdl)

if keep_flying == 0
    cum_out = cum_in + mdl.T;
else
    cum_out = 0;
end

if cum_out > ctr2.safety.land.T || landing_in == 1
    landing_out = 1;
else 
    landing_out = 0;
end

end

== matlab function controller13_jumping/Measurement manager 2/envelope//voltage check ==
  data: x input; keep_flying output size=1; y input; z input; ctr2 parameter
function keep_flying  = fcn(x,y,z,ctr2)

if abs(x)>ctr2.safety.land.xmax || abs(y)>ctr2.safety.land.ymax || abs(z)>ctr2.safety.land.zmax
    keep_flying = 0;
% elseif voltage(1) > ctr.safety.land.volt
%     keep_flying = 0;    
else
    keep_flying = 1;
end

end

== matlab function controller13_jumping/Measurement manager 2/safety check system/MATLAB Function ==
  data: keep_flying input; en_in input; en_out output size=1; cum_in input; cum_out output size=1; ctr2 parameter; mdl parameter
function [en_out, cum_out] = fcn(keep_flying, en_in, cum_in, ctr2, mdl)

if keep_flying == 0
    cum_out = cum_in + mdl.T;
else
    cum_out = 0;
end

if cum_out > ctr2.safety.T || en_in == 0
    en_out = 0;
else 
    en_out = 1;
end

end

== matlab function controller13_jumping/Measurement manager 2/safety check system/envelope check ==
  data: x input; en output; y input; z input; ctr2 parameter
function en  = fcn(x,y,z, ctr2)

if abs(x)>ctr2.safety.enableZone.xmax || abs(y)>ctr2.safety.enableZone.ymax || abs(z)>ctr2.safety.enableZone.zmax
    en = 0;
else
    en = 1;
end

end

== matlab function controller13_jumping/Measurement manager 2/safety check system/landing condition/landing_cond ==
  data: alt input; en output; time_cond input; ctr2 parameter
function en = fcn(alt,time_cond,ctr2)
%#codegen
if ( (time_cond<0) | (alt>ctr2.landing.height) )
    en = 1;
else
    en = 0;
end
en=1;
end
% this lands the robot if the flight time is more than mdl.i_delay+2 and
% the robot is still on the ground.

== matlab function controller13_jumping/Measurement manager 2/safety check system/voltage check ==
  data: voltage input; en output; ctr2 parameter
function en  = fcn(voltage, ctr2)

if sum(voltage>ctr2.safety.volt) > 0
    en = 0;
else
    en = 1;
end

end

== matlab function controller13_jumping/Measurement manager 2/voltage check ==
  data: voltage input; keep_flying output size=1; ctr2 parameter
function keep_flying  = fcn(voltage, ctr2)

% if voltage(1)>ctr.safety.land.volt || voltage(2)>ctr.safety.land.volt || voltage(3)>ctr.safety.land.volt || voltage(4)>ctr.safety.land.volt

if sum(voltage>ctr2.safety.land.volt)>0
    keep_flying = 0;
else
    keep_flying = 1;
end

end

== matlab function controller13_jumping/Jumping Simulation/power_distribution_1 ==
  data: thrust output; roll_arm input; pitch_arm input; motor_thrust input; torque output
function [thrust, torque] = fcn(roll_arm, pitch_arm, motor_thrust)

% motor_thrust is in mgf
torque_x_mgfm = (- motor_thrust(1) + motor_thrust(2) ...
                 + motor_thrust(3) - motor_thrust(4)) * roll_arm; % (mgf*m)
torque_y_mgfm = (- motor_thrust(1) - motor_thrust(2) ...
                 + motor_thrust(3) + motor_thrust(4)) * pitch_arm; % (mgf*m)
thrust_mgf    = (+ motor_thrust(1) + motor_thrust(2) ...
                 + motor_thrust(3) + motor_thrust(4)); % (mgf)        

% convert mgf to N (mgf*m & N*m)
torque = [torque_x_mgfm; torque_y_mgfm; 0] * 9.81e-6; %(N*m)
thrust = thrust_mgf * 9.81e-6; % (N)

% ==== original code ====
% r = torque(1) / roll_arm;
% p = torque(2) / pitch_arm; % (mgf) = (mgf*m) / (m)
% 
% att = [
%     - r - p;
%     + r - p;
%     + r + p;
%     - r + p]; % (mgf)
% 
% min_t = min(att);
% 
% if (thrust < - min_t)
%     thrust = - min_t; 
% end
%     
% m1 = thrust + att(1); % (mgf)
% m2 = thrust + att(2); % (mgf)
% m3 = thrust + att(3); % (mgf)
% m4 = thrust + att(4); % (mgf)
% 
% 
% motors_thrust = [m1; m2; m3; m4]; % (mgf)
% 
% return;
end

== matlab function controller13_jumping/Subsystem3/MATLAB Function ==
  data: u_x input; roll output; u_y input; yaw input; pitch output
function [roll, pitch] = fcn(u_x, u_y, yaw)

pitch = (u_x * cos(yaw) + u_y * sin(yaw));
roll = - (u_y * cos(yaw) - u_x * sin(yaw));

== matlab function controller13_jumping/Subsystem6/Subsystem5/Rotation Matrix ==
  data: euler_angles input; R output
function R = fcn(euler_angles)
%#codegen

eu_x = euler_angles(1);
eu_y = euler_angles(2);
eu_z = euler_angles(3);

R = [cos(eu_y)*cos(eu_z); -cos(eu_y)*sin(eu_z); sin(eu_y); ...
    cos(eu_x)*sin(eu_z)+sin(eu_x)*sin(eu_y)*cos(eu_z); cos(eu_x)*cos(eu_z)-sin(eu_x)*sin(eu_y)*sin(eu_z); -sin(eu_x)*cos(eu_y); ...
    sin(eu_x)*sin(eu_z)-cos(eu_x)*sin(eu_y)*cos(eu_z); sin(eu_x)*cos(eu_z)+cos(eu_x)*sin(eu_y)*sin(eu_z); cos(eu_x)*cos(eu_y)];


end

% R is 9x1

% Pakpong was using "XYZ" convention, which seems to be the same as Vicon

== matlab function controller13_jumping/Subsystem6/Subsystem5/Rotation Matrix1 ==
  data: R input; Rdot input; w output
function w  = fcn(R,Rdot)
%#codegen
w = zeros(3,1);
w(1) = R(3)*Rdot(2) + R(6)*Rdot(5) + R(9)*Rdot(8);
w(2) = R(1)*Rdot(3) + R(4)*Rdot(6) + R(7)*Rdot(9);
w(3) = R(2)*Rdot(1) + R(5)*Rdot(4) + R(8)*Rdot(7);

% w = R^T * dot(R)

end

== matlab function controller13_jumping/jumping_state_tracker ==
  data: controller_trigger output; foot_height output; p input; p_dot input; rotm input; jumping_state output; leg_length input; foot_alitutde_threshold input; jumping_state_old input
function [controller_trigger, foot_height, jumping_state] = fcn(p, p_dot, rotm, leg_length, foot_alitutde_threshold, jumping_state_old)

p_foot = p + rotm * [0;0; -leg_length];

controller_trigger = false;

% 1 for falling phase, 2 for jumping phase, 3 for climbing phase, 0 for flight mode
jumping_state = jumping_state_old;
if p_foot(3) < foot_alitutde_threshold
    jumping_state = 2;  % stance phase
elseif p_dot(3) > 0.3 && jumping_state_old == 2
    jumping_state = 3;  % climbing phase
elseif p_dot(3) < 0.05 && jumping_state_old == 3
    jumping_state = 1;  % falling phase
    controller_trigger = true;
end

foot_height = p_foot(3);
return;
end

== matlab function controller13_jumping/power_distribution_2 ==
  data: roll_arm input; pitch_arm input; torque input; motors_thrust output; thrust input
function motors_thrust = fcn(roll_arm, pitch_arm, torque, thrust)

r = torque(1) / roll_arm;
p = torque(2) / pitch_arm;

% m1 = thrust - r - p;
% m2 = thrust + r - p;
% m3 = thrust + r + p;
% m4 = thrust - r + p;
att = [
    - r - p;
    + r - p;
    + r + p;
    - r + p];

min_t = min(att);

if (thrust < - min_t)
    thrust = - min_t; 
end
    
m1 = thrust + att(1);
m2 = thrust + att(2);
m3 = thrust + att(3);
m4 = thrust + att(4);


motors_thrust = [m1; m2; m3; m4];

return;
end

== matlab function controller13_jumping/landing attitude controller/inverse_jumping_model ==
  data: p_dot_landing input; landing_attitude_z_b output; p_dot_takeoff input; k2 input
function landing_attitude_z_b = fcn(p_dot_landing, p_dot_takeoff, k2)

p_dot_ld = norm(p_dot_landing);
v_surface = cross(-p_dot_landing, p_dot_takeoff);
v_surface_norm = norm(v_surface);

if v_surface_norm < 0.000001
    v_surface(1) = 1;
    v_surface(2) = 0;
    v_surface(3) = 0;
else
    v_surface = v_surface/v_surface_norm;
end
theta_v = atan2(v_surface_norm, dot(-p_dot_landing, p_dot_takeoff));

%% in plane jumping model
theta_l = theta_v / k2;
% p_dot_tk = p_dot_ld * k3;
% theta_t = theta_l * k1;
% beta = theta_t - theta_l;

axang = [v_surface', theta_l];
landing_attitude_z_b = axang2rotm(axang) * (-p_dot_landing) / p_dot_ld;

== matlab function controller13_jumping/landing attitude controller/jumping_planning ==
  data: g input; velocity_limit_ratio input; p_dot_TK input; p_landing input; desired_x input; desired_y input; jumping_altitude input; takeoff_velocity output; mdl parameter
function takeoff_velocity = fcn(g, velocity_limit_ratio, ...
    p_dot_TK, p_landing,...
    desired_x, desired_y, jumping_altitude, mdl)

time_climb = sqrt(2*jumping_altitude/g);
time_fall = time_climb;
time_plan = time_climb + time_fall;
u_x = (desired_x - p_landing(1))/time_plan;
u_y = (desired_y - p_landing(2))/time_plan;
norm_v = sqrt(u_x*u_x + u_y*u_y);

predicted_takeoff_speed = p_dot_TK;

lateral_velocity_limit = predicted_takeoff_speed*velocity_limit_ratio;
if norm_v > lateral_velocity_limit
    u_x = lateral_velocity_limit * u_x/norm_v;
    u_y = lateral_velocity_limit * u_y/norm_v;
end
u_x = u_x * mdl.predicted_x_factor;
u_y = u_y * mdl.predicted_y_factor;

takeoff_velocity = [u_x; u_y; g*time_climb];
end
